simulink model "SecRwRtStLgrstInwdOtwdIsPosChk"  (R2024b)
settings: Solver=FixedStepDiscrete  StartTime=0.0  StopTime=10.0  FixedStep=0.01  RelTol=1e-3
undefined symbols (not defined in the file or in its folder): KeSMSuSecRwStLegrestInOutPosDelta_Val, KeSMSuSecRwStLegrestInOutPosTolr_Val
libraries: StIsPosChkLib x18, simulink x8
(part 1 of 2)
settings Model: Creator=sn2xws  LastModifiedBy=sn55gm
settings Model: ModifiedHistory=|
  | 2023.8.1 V2.0.0 CR421790 增加模式21-26
  | 2023.9.14 V2.1.0 Bug 540886 修改模式判断到位的条件为10ms周期计算
  | 2024.5.8 V3.0.0 557 eze 模式变更
  | 2024.7.9 V3.0.1 557模式流程V1.9
  | 2024.8.15 V3.0.2 智享模式需要计算目标位置，不能直接判断到位置，posalready赋值0
  | 2024.8.29 V3.0.3智享VIP目标位置用了4s问题修复
  | 2024.9.5 V3.0.4 新增Md56，注释不用的模式
  | 2024.10.14 V3.0.5 新增Md57，Md58
  | 2024.11.27 V3.0.6 Md57运行时，不能直接判断到位置
  | 25.7.7 V3.13.0 新增Md61 Md62 Md30 Md31
  | 25.10.30 V3.13.1 mode30标定修改
settings SolverCC: AlgebraicLoopSolver=TrustRegion
settings DataIOCC: SaveFormat=StructureWithTime  ReturnWorkspaceOutputs=off
settings OptimizationCC: DefaultParameterBehavior=Inlined  EnhancedBackFolding=on  PassReuseOutputArgsAs=Individual arguments  ZeroExternalMemoryAtStartup=off  ZeroInternalMemoryAtStartup=off  OptimizeBlockOrder=speed  DifferentSizesBufferReuse=on  OptimizationCustomize=off  EfficientTunableParamExpr=on
settings DebuggingCC: ParameterTunabilityLossMsg=error  UnconnectedInputMsg=warning  UnconnectedOutputMsg=warning  UnconnectedLineMsg=warning  ArithmeticOperatorsInVariantConditions=warning
settings ModelReferenceCC: EnableRefExpFcnMdlSchedulingChecks=on  ModelReferenceNumInstancesAllowed=Single
settings SFSimCC: MATLABDynamicMemAlloc=off  CustomCodeUndefinedFunction=UseInterfaceOnly
settings RTWCC: Description=AUTOSAR  SystemTargetFile=autosar.tlc  GenCodeOnly=on  TemplateMakefile=ert_default_tmf  GenerateReport=on  IncludeHyperlinkInReport=on  LaunchReport=on  DataTypeReplacement=CDataTypesFixedWidth  GenerateTraceInfo=on  GenerateTraceReport=on  GenerateTraceReportSl=on  GenerateTraceReportSf=on  GenerateTraceReportEml=on  GPUComputeCapability=3.5
settings CodeAppCC: ForceParamTrailComments=on  IgnoreCustomStorageClasses=off  OperatorAnnotations=on  SimulinkDataObjDesc=on  SFDataObjDesc=on  InsertBlockDesc=on
settings STFCustomTargetCC: TargetLangStandard=C99 (ISO)  MultiwordLength=256  ParMdlRefBuildCompliant=on  CompOptLevelCompliant=on  IncludeMdlTerminateFcn=off  CombineOutputUpdateFcns=on  SuppressErrorStatus=on  ERTCustomFileBanners=on  SupportNonFinite=off  SupportComplex=off  SupportContinuousTime=off  SupportNonInlinedSFcns=off  RemoveResetFunc=on  MATLABClassNameForMDSCustomization=Simulink.SoftwareTarget.ERTCustomization  AutosarCompliant=on  UseToolchainInfoCompliant=on  LookupTableObjectStructAxisOrder=2,1,3,4,...  LUTObjectStructOrderEvenSpacing=Size,Table,Breakpoints  SystemTargetFile=autosar.tlc
settings ERTTargetCC: TargetLangStandard=C99 (ISO)  ConcurrentExecutionCompliant=off  IncludeMdlTerminateFcn=off  SuppressErrorStatus=on  SupportNonFinite=off  SupportComplex=off  ModelStepFunctionPrototypeControlCompliant=off  CPPClassGenCompliant=off  AutosarCompliant=on  LookupTableObjectStructAxisOrder=2,1,3,4,...  LUTObjectStructOrderEvenSpacing=Size,Table,Breakpoints  ERTCustomFileTemplate=example_file_process.tlc  ERTFilePackagingFormat=Compact  BooleanTrueId=TRUE  BooleanFalseId=FALSE  DynamicArrayContainerType=coder::array

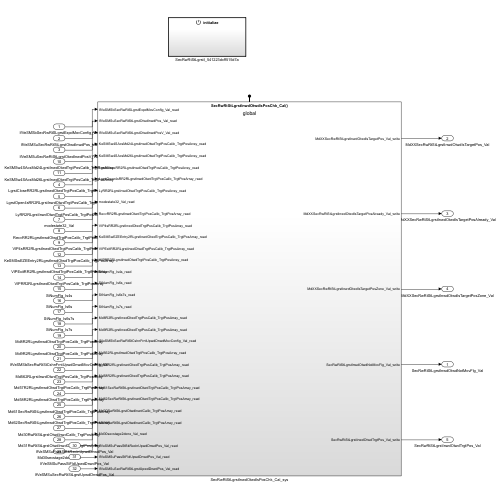
[thumbnail: Simulink's stored preview of the top-level diagram]
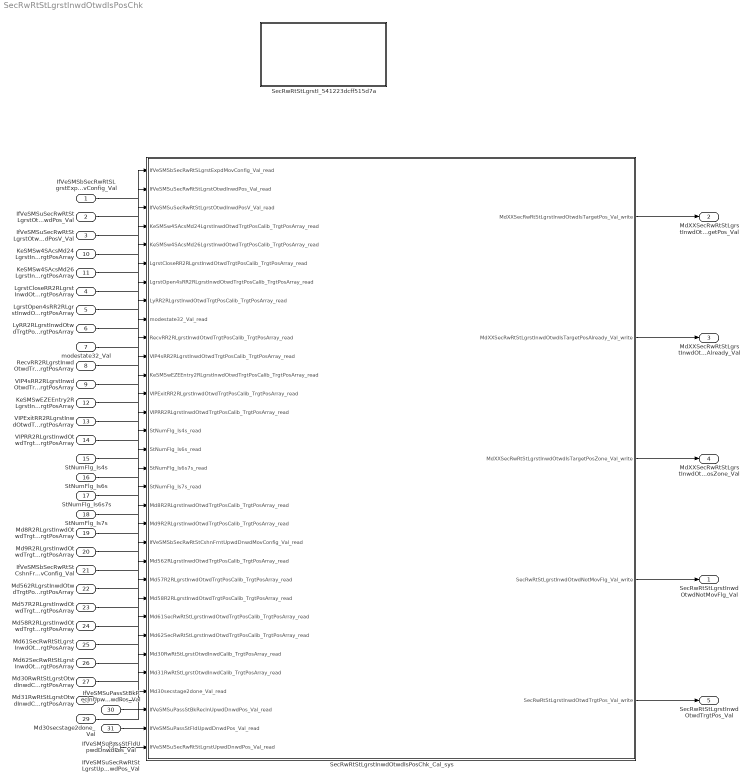
== system SecRwRtStLgrstInwdOtwdIsPosChk ==
  IfVeSMSbSecRwRtSLgrstExpdMovConfig_Val : Inport  OutDataTypeStr=boolean  PortDimensions=1
  IfVeSMSuSecRwRtStLgrstOtwdInwdPos_Val : Inport  Port=2  OutDataTypeStr=uint16  PortDimensions=1
  IfVeSMSuSecRwRtStLgrstOtwdInwdPosV_Val : Inport  Port=3  OutDataTypeStr=boolean  PortDimensions=1
  LgrstCloseRR2RLgrstInwdOtwdTrgtPosCalib_TrgtPosArray : Inport  Description=|  Port=4  OutDataTypeStr=uint16  PortDimensions=3
      | 0:Pos
      | 1:Max
      | 2:Min
  LgrstOpen4sRR2RLgrstInwdOtwdTrgtPosCalib_TrgtPosArray : Inport  Description=|  Port=5  OutDataTypeStr=uint16  PortDimensions=3
      | 0:Pos
      | 1:Max
      | 2:Min
  LyRR2RLgrstInwdOtwdTrgtPosCalib_TrgtPosArray : Inport  Description=|  Port=6  OutDataTypeStr=uint16  PortDimensions=3
      | 0:Pos
      | 1:Max
      | 2:Min
  modestate32_Val : Inport  Port=7  OutDataTypeStr=uint32  PortDimensions=1
  RecvRR2RLgrstInwdOtwdTrgtPosCalib_TrgtPosArray : Inport  Description=|  Port=8  OutDataTypeStr=uint16  PortDimensions=3
      | 0:Pos
      | 1:Max
      | 2:Min
  VIP4sRR2RLgrstInwdOtwdTrgtPosCalib_TrgtPosArray : Inport  Description=|  Port=9  OutDataTypeStr=uint16  PortDimensions=3
      | 0:Pos
      | 1:Max
      | 2:Min
  KeSMSw4SAcsMd24LgrstInwdOtwdTrgtPosCalib_TrgtPosArray : Inport  Description=|  Port=10  OutDataTypeStr=uint16  PortDimensions=3
      | 0:Pos
      | 1:Max
      | 2:Min
  KeSMSw4SAcsMd26LgrstInwdOtwdTrgtPosCalib_TrgtPosArray : Inport  Description=|  Port=11  OutDataTypeStr=uint16  PortDimensions=3
      | 0:Pos
      | 1:Max
      | 2:Min
  KeSMSwEZEEntry2RLgrstInwdOtwdTrgtPosCalib_TrgtPosArray : Inport  Description=|  Port=12  OutDataTypeStr=uint16  PortDimensions=3
      | 0:Pos
      | 1:Max
      | 2:Min
  VIPExitRR2RLgrstInwdOtwdTrgtPosCalib_TrgtPosArray : Inport  Description=|  Port=13  OutDataTypeStr=uint16  PortDimensions=3
      | 0:Pos
      | 1:Max
      | 2:Min
  VIPRR2RLgrstInwdOtwdTrgtPosCalib_TrgtPosArray : Inport  Description=|  Port=14  OutDataTypeStr=uint16  PortDimensions=3
      | 0:Pos
      | 1:Max
      | 2:Min
  StNumFlg_Is4s : Inport  Port=15  OutDataTypeStr=boolean  PortDimensions=1
  StNumFlg_Is6s : Inport  Port=16  OutDataTypeStr=boolean  PortDimensions=1
  StNumFlg_Is6s7s : Inport  Port=17  OutDataTypeStr=boolean  PortDimensions=1
  StNumFlg_Is7s : Inport  Port=18  OutDataTypeStr=boolean  PortDimensions=1
  Md8R2RLgrstInwdOtwdTrgtPosCalib_TrgtPosArray : Inport  Description=|  Port=19  OutDataTypeStr=uint16  PortDimensions=3
      | 0:Pos
      | 1:Max
      | 2:Min
  Md9R2RLgrstInwdOtwdTrgtPosCalib_TrgtPosArray : Inport  Description=|  Port=20  OutDataTypeStr=uint16  PortDimensions=3
      | 0:Pos
      | 1:Max
      | 2:Min
  IfVeSMSbSecRwRtStCshnFrntUpwdDnwdMovConfig_Val : Inport  Port=21  OutDataTypeStr=boolean  PortDimensions=1
  Md562RLgrstInwdOtwdTrgtPosCalib_TrgtPosArray : Inport  Description=|  Port=22  OutDataTypeStr=uint16  PortDimensions=3
      | 0:Pos
      | 1:Max
      | 2:Min
  Md57R2RLgrstInwdOtwdTrgtPosCalib_TrgtPosArray : Inport  Description=|  Port=23  OutDataTypeStr=uint16  PortDimensions=3
      | 0:Pos
      | 1:Max
      | 2:Min
  Md58R2RLgrstInwdOtwdTrgtPosCalib_TrgtPosArray : Inport  Description=|  Port=24  OutDataTypeStr=uint16  PortDimensions=3
      | 0:Pos
      | 1:Max
      | 2:Min
  Md61SecRwRtStLgrstInwdOtwdTrgtPosCalib_TrgtPosArray : Inport  Description=|  Port=25  OutDataTypeStr=uint16  PortDimensions=3
      | 0:Pos
      | 1:Max
      | 2:Min
  Md62SecRwRtStLgrstInwdOtwdTrgtPosCalib_TrgtPosArray : Inport  Description=|  Port=26  OutDataTypeStr=uint16  PortDimensions=3
      | 0:Pos
      | 1:Max
      | 2:Min
  Md30RwRtStLgrstOtwdInwdCalib_TrgtPosArray : Inport  Description=|  Port=27  OutDataTypeStr=uint16  PortDimensions=3
      | 0:Pos
      | 1:Max
      | 2:Min
  Md31RwRtStLgrstOtwdInwdCalib_TrgtPosArray : Inport  Description=|  Port=28  OutDataTypeStr=uint16  PortDimensions=3
      | 0:Pos
      | 1:Max
      | 2:Min
  Md30secstage2done_Val : Inport  Port=29  OutDataTypeStr=uint8  PortDimensions=1
  IfVeSMSuPassStBkReclnUpwdDnwdPos_Val : Inport  Port=30  OutDataTypeStr=uint16  PortDimensions=1
  IfVeSMSuPassStFldUpwdDnwdPos_Val : Inport  Port=31  OutDataTypeStr=uint16  PortDimensions=1
  IfVeSMSuSecRwRtStLgrstUpwdDnwdPos_Val : Inport  Port=32  OutDataTypeStr=uint16  PortDimensions=1
  SecRwRtStLgrstI_541223dcff515d7a : Subsystem
  SecRwRtStLgrstInwdOtwdIsPosChk_Cal_sys : Subsystem
  SecRwRtStLgrstInwdOtwdNotMovFlg_Val : Outport  OutDataTypeStr=boolean  PortDimensions=1  VectorParamsAs1DForOutWhenUnconnected=off
  MdXXSecRwRtStLgrstInwdOtwdIsTargetPos_Val : Outport  Port=2  OutDataTypeStr=uint32  PortDimensions=1  VectorParamsAs1DForOutWhenUnconnected=off
  MdXXSecRwRtStLgrstInwdOtwdIsTargetPosAlready_Val : Outport  Port=3  OutDataTypeStr=uint32  PortDimensions=1  VectorParamsAs1DForOutWhenUnconnected=off
  MdXXSecRwRtStLgrstInwdOtwdIsTargetPosZone_Val : Outport  Port=4  OutDataTypeStr=uint32  PortDimensions=1  VectorParamsAs1DForOutWhenUnconnected=off
  SecRwRtStLgrstInwdOtwdTrgtPos_Val : Outport  Port=5  OutDataTypeStr=uint16  PortDimensions=1  VectorParamsAs1DForOutWhenUnconnected=off
  wires:
  IfVeSMSbSecRwRtSLgrstExpdMovConfig_Val/1 -> SecRwRtStLgrstInwdOtwdIsPosChk_Cal_sys/1(IfVeSMSbSecRwRtSLgrstExpdMovConfig_Val_read)
  IfVeSMSuSecRwRtStLgrstOtwdInwdPos_Val/1 -> SecRwRtStLgrstInwdOtwdIsPosChk_Cal_sys/2(IfVeSMSuSecRwRtStLgrstOtwdInwdPos_Val_read)
  IfVeSMSuSecRwRtStLgrstOtwdInwdPosV_Val/1 -> SecRwRtStLgrstInwdOtwdIsPosChk_Cal_sys/3(IfVeSMSuSecRwRtStLgrstOtwdInwdPosV_Val_read)
  LgrstCloseRR2RLgrstInwdOtwdTrgtPosCalib_TrgtPosArray/1 -> SecRwRtStLgrstInwdOtwdIsPosChk_Cal_sys/6(LgrstCloseRR2RLgrstInwdOtwdTrgtPosCalib_TrgtPosArray_read)
  LgrstOpen4sRR2RLgrstInwdOtwdTrgtPosCalib_TrgtPosArray/1 -> SecRwRtStLgrstInwdOtwdIsPosChk_Cal_sys/7(LgrstOpen4sRR2RLgrstInwdOtwdTrgtPosCalib_TrgtPosArray_read)
  LyRR2RLgrstInwdOtwdTrgtPosCalib_TrgtPosArray/1 -> SecRwRtStLgrstInwdOtwdIsPosChk_Cal_sys/8(LyRR2RLgrstInwdOtwdTrgtPosCalib_TrgtPosArray_read)
  RecvRR2RLgrstInwdOtwdTrgtPosCalib_TrgtPosArray/1 -> SecRwRtStLgrstInwdOtwdIsPosChk_Cal_sys/10(RecvRR2RLgrstInwdOtwdTrgtPosCalib_TrgtPosArray_read)
  VIP4sRR2RLgrstInwdOtwdTrgtPosCalib_TrgtPosArray/1 -> SecRwRtStLgrstInwdOtwdIsPosChk_Cal_sys/11(VIP4sRR2RLgrstInwdOtwdTrgtPosCalib_TrgtPosArray_read)
  SecRwRtStLgrstInwdOtwdIsPosChk_Cal_sys/1(MdXXSecRwRtStLgrstInwdOtwdIsTargetPos_Val_write) -> MdXXSecRwRtStLgrstInwdOtwdIsTargetPos_Val/1
  SecRwRtStLgrstInwdOtwdIsPosChk_Cal_sys/2(MdXXSecRwRtStLgrstInwdOtwdIsTargetPosAlready_Val_write) -> MdXXSecRwRtStLgrstInwdOtwdIsTargetPosAlready_Val/1
  SecRwRtStLgrstInwdOtwdIsPosChk_Cal_sys/3(MdXXSecRwRtStLgrstInwdOtwdIsTargetPosZone_Val_write) -> MdXXSecRwRtStLgrstInwdOtwdIsTargetPosZone_Val/1
  SecRwRtStLgrstInwdOtwdIsPosChk_Cal_sys/4(SecRwRtStLgrstInwdOtwdNotMovFlg_Val_write) -> SecRwRtStLgrstInwdOtwdNotMovFlg_Val/1
  SecRwRtStLgrstInwdOtwdIsPosChk_Cal_sys/5(SecRwRtStLgrstInwdOtwdTrgtPos_Val_write) -> SecRwRtStLgrstInwdOtwdTrgtPos_Val/1
  KeSMSw4SAcsMd24LgrstInwdOtwdTrgtPosCalib_TrgtPosArray/1 -> SecRwRtStLgrstInwdOtwdIsPosChk_Cal_sys/4(KeSMSw4SAcsMd24LgrstInwdOtwdTrgtPosCalib_TrgtPosArray_read)
  KeSMSw4SAcsMd26LgrstInwdOtwdTrgtPosCalib_TrgtPosArray/1 -> SecRwRtStLgrstInwdOtwdIsPosChk_Cal_sys/5(KeSMSw4SAcsMd26LgrstInwdOtwdTrgtPosCalib_TrgtPosArray_read)
  modestate32_Val/1 -> SecRwRtStLgrstInwdOtwdIsPosChk_Cal_sys/9(modestate32_Val_read)
  KeSMSwEZEEntry2RLgrstInwdOtwdTrgtPosCalib_TrgtPosArray/1 -> SecRwRtStLgrstInwdOtwdIsPosChk_Cal_sys/12(KeSMSwEZEEntry2RLgrstInwdOtwdTrgtPosCalib_TrgtPosArray_read)
  VIPExitRR2RLgrstInwdOtwdTrgtPosCalib_TrgtPosArray/1 -> SecRwRtStLgrstInwdOtwdIsPosChk_Cal_sys/13(VIPExitRR2RLgrstInwdOtwdTrgtPosCalib_TrgtPosArray_read)
  VIPRR2RLgrstInwdOtwdTrgtPosCalib_TrgtPosArray/1 -> SecRwRtStLgrstInwdOtwdIsPosChk_Cal_sys/14(VIPRR2RLgrstInwdOtwdTrgtPosCalib_TrgtPosArray_read)
  StNumFlg_Is4s/1 -> SecRwRtStLgrstInwdOtwdIsPosChk_Cal_sys/15(StNumFlg_Is4s_read)
  StNumFlg_Is6s/1 -> SecRwRtStLgrstInwdOtwdIsPosChk_Cal_sys/16(StNumFlg_Is6s_read)
  StNumFlg_Is6s7s/1 -> SecRwRtStLgrstInwdOtwdIsPosChk_Cal_sys/17(StNumFlg_Is6s7s_read)
  StNumFlg_Is7s/1 -> SecRwRtStLgrstInwdOtwdIsPosChk_Cal_sys/18(StNumFlg_Is7s_read)
  Md8R2RLgrstInwdOtwdTrgtPosCalib_TrgtPosArray/1 -> SecRwRtStLgrstInwdOtwdIsPosChk_Cal_sys/19(Md8R2RLgrstInwdOtwdTrgtPosCalib_TrgtPosArray_read)
  Md9R2RLgrstInwdOtwdTrgtPosCalib_TrgtPosArray/1 -> SecRwRtStLgrstInwdOtwdIsPosChk_Cal_sys/20(Md9R2RLgrstInwdOtwdTrgtPosCalib_TrgtPosArray_read)
  IfVeSMSbSecRwRtStCshnFrntUpwdDnwdMovConfig_Val/1 -> SecRwRtStLgrstInwdOtwdIsPosChk_Cal_sys/21(IfVeSMSbSecRwRtStCshnFrntUpwdDnwdMovConfig_Val_read)
  Md562RLgrstInwdOtwdTrgtPosCalib_TrgtPosArray/1 -> SecRwRtStLgrstInwdOtwdIsPosChk_Cal_sys/22(Md562RLgrstInwdOtwdTrgtPosCalib_TrgtPosArray_read)
  Md57R2RLgrstInwdOtwdTrgtPosCalib_TrgtPosArray/1 -> SecRwRtStLgrstInwdOtwdIsPosChk_Cal_sys/23(Md57R2RLgrstInwdOtwdTrgtPosCalib_TrgtPosArray_read)
  Md58R2RLgrstInwdOtwdTrgtPosCalib_TrgtPosArray/1 -> SecRwRtStLgrstInwdOtwdIsPosChk_Cal_sys/24(Md58R2RLgrstInwdOtwdTrgtPosCalib_TrgtPosArray_read)
  Md61SecRwRtStLgrstInwdOtwdTrgtPosCalib_TrgtPosArray/1 -> SecRwRtStLgrstInwdOtwdIsPosChk_Cal_sys/25(Md61SecRwRtStLgrstInwdOtwdTrgtPosCalib_TrgtPosArray_read)
  Md62SecRwRtStLgrstInwdOtwdTrgtPosCalib_TrgtPosArray/1 -> SecRwRtStLgrstInwdOtwdIsPosChk_Cal_sys/26(Md62SecRwRtStLgrstInwdOtwdTrgtPosCalib_TrgtPosArray_read)
  Md30RwRtStLgrstOtwdInwdCalib_TrgtPosArray/1 -> SecRwRtStLgrstInwdOtwdIsPosChk_Cal_sys/27(Md30RwRtStLgrstOtwdInwdCalib_TrgtPosArray_read)
  Md31RwRtStLgrstOtwdInwdCalib_TrgtPosArray/1 -> SecRwRtStLgrstInwdOtwdIsPosChk_Cal_sys/28(Md31RwRtStLgrstOtwdInwdCalib_TrgtPosArray_read)
  Md30secstage2done_Val/1 -> SecRwRtStLgrstInwdOtwdIsPosChk_Cal_sys/29(Md30secstage2done_Val_read)
  IfVeSMSuPassStBkReclnUpwdDnwdPos_Val/1 -> SecRwRtStLgrstInwdOtwdIsPosChk_Cal_sys/30(IfVeSMSuPassStBkReclnUpwdDnwdPos_Val_read)
  IfVeSMSuPassStFldUpwdDnwdPos_Val/1 -> SecRwRtStLgrstInwdOtwdIsPosChk_Cal_sys/31(IfVeSMSuPassStFldUpwdDnwdPos_Val_read)
  IfVeSMSuSecRwRtStLgrstUpwdDnwdPos_Val/1 -> SecRwRtStLgrstInwdOtwdIsPosChk_Cal_sys/32(IfVeSMSuSecRwRtStLgrstUpwdDnwdPos_Val_read)

== system SecRwRtStLgrstInwdOtwdIsPosChk/SecRwRtStLgrstI_541223dcff515d7a ==
  note: Added blocks
  note: Added blocks
  Event Listener : EventListener  EventName=reset
  PA_KeSMSuSecRwStLegrestInOutPosDelta_Val : Constant  Value=KeSMSuSecRwStLegrestInOutPosDelta_Val
  PA_KeSMSuSecRwStLegrestInOutPosTolr_Val : Constant  Value=KeSMSuSecRwStLegrestInOutPosTolr_Val
  Terminator_1 : Terminator
  Terminator_2 : Terminator
  wires:
  PA_KeSMSuSecRwStLegrestInOutPosDelta_Val/1 -> Terminator_1/1
  PA_KeSMSuSecRwStLegrestInOutPosTolr_Val/1 -> Terminator_2/1

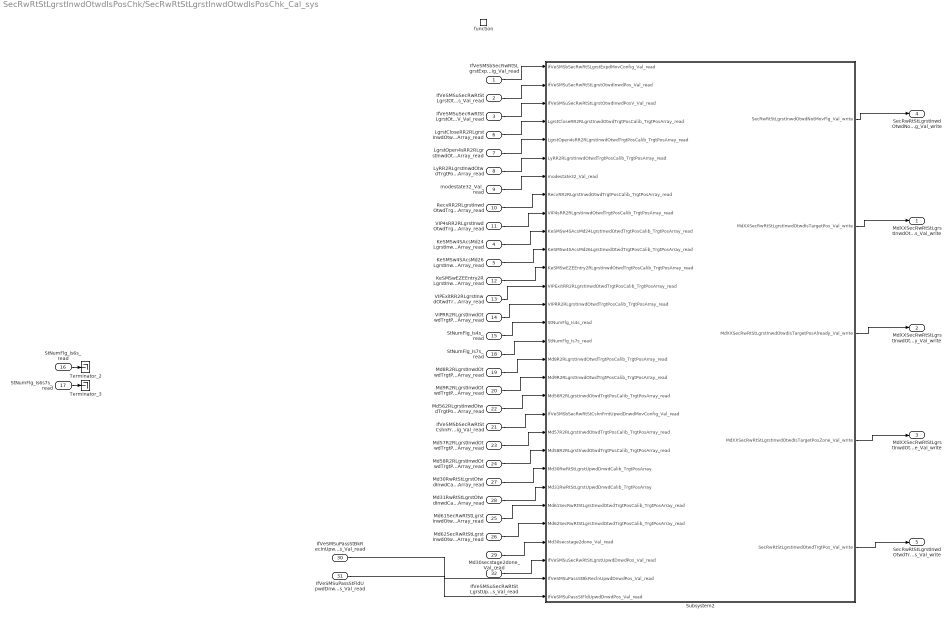
== system SecRwRtStLgrstInwdOtwdIsPosChk/SecRwRtStLgrstInwdOtwdIsPosChk_Cal_sys ==
  IfVeSMSbSecRwRtSLgrstExpdMovConfig_Val_read : Inport
  IfVeSMSuSecRwRtStLgrstOtwdInwdPos_Val_read : Inport  Port=2
  IfVeSMSuSecRwRtStLgrstOtwdInwdPosV_Val_read : Inport  Port=3
  KeSMSw4SAcsMd24LgrstInwdOtwdTrgtPosCalib_TrgtPosArray_read : Inport  Port=4
  KeSMSw4SAcsMd26LgrstInwdOtwdTrgtPosCalib_TrgtPosArray_read : Inport  Port=5
  LgrstCloseRR2RLgrstInwdOtwdTrgtPosCalib_TrgtPosArray_read : Inport  Port=6
  LgrstOpen4sRR2RLgrstInwdOtwdTrgtPosCalib_TrgtPosArray_read : Inport  Port=7
  LyRR2RLgrstInwdOtwdTrgtPosCalib_TrgtPosArray_read : Inport  Port=8
  modestate32_Val_read : Inport  Port=9
  RecvRR2RLgrstInwdOtwdTrgtPosCalib_TrgtPosArray_read : Inport  Port=10
  VIP4sRR2RLgrstInwdOtwdTrgtPosCalib_TrgtPosArray_read : Inport  Port=11
  KeSMSwEZEEntry2RLgrstInwdOtwdTrgtPosCalib_TrgtPosArray_read : Inport  Port=12
  VIPExitRR2RLgrstInwdOtwdTrgtPosCalib_TrgtPosArray_read : Inport  Port=13
  VIPRR2RLgrstInwdOtwdTrgtPosCalib_TrgtPosArray_read : Inport  Port=14
  StNumFlg_Is4s_read : Inport  Port=15
  StNumFlg_Is6s_read : Inport  Port=16
  StNumFlg_Is6s7s_read : Inport  Port=17
  StNumFlg_Is7s_read : Inport  Port=18
  Md8R2RLgrstInwdOtwdTrgtPosCalib_TrgtPosArray_read : Inport  Port=19
  Md9R2RLgrstInwdOtwdTrgtPosCalib_TrgtPosArray_read : Inport  Port=20
  IfVeSMSbSecRwRtStCshnFrntUpwdDnwdMovConfig_Val_read : Inport  Port=21
  Md562RLgrstInwdOtwdTrgtPosCalib_TrgtPosArray_read : Inport  Port=22
  Md57R2RLgrstInwdOtwdTrgtPosCalib_TrgtPosArray_read : Inport  Port=23
  Md58R2RLgrstInwdOtwdTrgtPosCalib_TrgtPosArray_read : Inport  Port=24
  Md61SecRwRtStLgrstInwdOtwdTrgtPosCalib_TrgtPosArray_read : Inport  Port=25
  Md62SecRwRtStLgrstInwdOtwdTrgtPosCalib_TrgtPosArray_read : Inport  Port=26
  Md30RwRtStLgrstOtwdInwdCalib_TrgtPosArray_read : Inport  Port=27
  Md31RwRtStLgrstOtwdInwdCalib_TrgtPosArray_read : Inport  Port=28
  Md30secstage2done_Val_read : Inport  Port=29
  IfVeSMSuPassStBkReclnUpwdDnwdPos_Val_read : Inport  Port=30
  IfVeSMSuPassStFldUpwdDnwdPos_Val_read : Inport  Port=31
  IfVeSMSuSecRwRtStLgrstUpwdDnwdPos_Val_read : Inport  Port=32
  function : TriggerPort  TriggerType=function-call  IsSimulinkFunction=on  FunctionName=SecRwRtStLgrstInwdOtwdIsPosChk_Cal  VariantControl=(inherit)
  Subsystem2 : Subsystem
  Terminator_2 : Terminator
  Terminator_3 : Terminator
  MdXXSecRwRtStLgrstInwdOtwdIsTargetPos_Val_write : Outport  VectorParamsAs1DForOutWhenUnconnected=off
      settings: EnsureOutportIsVirtual=on
  MdXXSecRwRtStLgrstInwdOtwdIsTargetPosAlready_Val_write : Outport  Port=2  VectorParamsAs1DForOutWhenUnconnected=off
      settings: EnsureOutportIsVirtual=on
  MdXXSecRwRtStLgrstInwdOtwdIsTargetPosZone_Val_write : Outport  Port=3  VectorParamsAs1DForOutWhenUnconnected=off
      settings: EnsureOutportIsVirtual=on
  SecRwRtStLgrstInwdOtwdNotMovFlg_Val_write : Outport  Port=4  VectorParamsAs1DForOutWhenUnconnected=off
      settings: EnsureOutportIsVirtual=on
  SecRwRtStLgrstInwdOtwdTrgtPos_Val_write : Outport  Port=5  VectorParamsAs1DForOutWhenUnconnected=off
      settings: EnsureOutportIsVirtual=on
  wires:
  Subsystem2/1(SecRwRtStLgrstInwdOtwdNotMovFlg_Val_write) -> SecRwRtStLgrstInwdOtwdNotMovFlg_Val_write/1
  Subsystem2/2(MdXXSecRwRtStLgrstInwdOtwdIsTargetPos_Val_write) -> MdXXSecRwRtStLgrstInwdOtwdIsTargetPos_Val_write/1
  Subsystem2/3(MdXXSecRwRtStLgrstInwdOtwdIsTargetPosAlready_Val_write) -> MdXXSecRwRtStLgrstInwdOtwdIsTargetPosAlready_Val_write/1
  Subsystem2/4(MdXXSecRwRtStLgrstInwdOtwdIsTargetPosZone_Val_write) -> MdXXSecRwRtStLgrstInwdOtwdIsTargetPosZone_Val_write/1
  Subsystem2/5(SecRwRtStLgrstInwdOtwdTrgtPos_Val_write) -> SecRwRtStLgrstInwdOtwdTrgtPos_Val_write/1
  VIP4sRR2RLgrstInwdOtwdTrgtPosCalib_TrgtPosArray_read/1 -> Subsystem2/9(VIP4sRR2RLgrstInwdOtwdTrgtPosCalib_TrgtPosArray_read)
  modestate32_Val_read/1 -> Subsystem2/7(modestate32_Val_read)
  RecvRR2RLgrstInwdOtwdTrgtPosCalib_TrgtPosArray_read/1 -> Subsystem2/8(RecvRR2RLgrstInwdOtwdTrgtPosCalib_TrgtPosArray_read)
  KeSMSw4SAcsMd24LgrstInwdOtwdTrgtPosCalib_TrgtPosArray_read/1 -> Subsystem2/10(KeSMSw4SAcsMd24LgrstInwdOtwdTrgtPosCalib_TrgtPosArray_read)
  KeSMSw4SAcsMd26LgrstInwdOtwdTrgtPosCalib_TrgtPosArray_read/1 -> Subsystem2/11(KeSMSw4SAcsMd26LgrstInwdOtwdTrgtPosCalib_TrgtPosArray_read)
  IfVeSMSbSecRwRtSLgrstExpdMovConfig_Val_read/1 -> Subsystem2/1(IfVeSMSbSecRwRtSLgrstExpdMovConfig_Val_read)
  IfVeSMSuSecRwRtStLgrstOtwdInwdPos_Val_read/1 -> Subsystem2/2(IfVeSMSuSecRwRtStLgrstOtwdInwdPos_Val_read)
  IfVeSMSuSecRwRtStLgrstOtwdInwdPosV_Val_read/1 -> Subsystem2/3(IfVeSMSuSecRwRtStLgrstOtwdInwdPosV_Val_read)
  LgrstCloseRR2RLgrstInwdOtwdTrgtPosCalib_TrgtPosArray_read/1 -> Subsystem2/4(LgrstCloseRR2RLgrstInwdOtwdTrgtPosCalib_TrgtPosArray_read)
  LgrstOpen4sRR2RLgrstInwdOtwdTrgtPosCalib_TrgtPosArray_read/1 -> Subsystem2/5(LgrstOpen4sRR2RLgrstInwdOtwdTrgtPosCalib_TrgtPosArray_read)
  LyRR2RLgrstInwdOtwdTrgtPosCalib_TrgtPosArray_read/1 -> Subsystem2/6(LyRR2RLgrstInwdOtwdTrgtPosCalib_TrgtPosArray_read)
  KeSMSwEZEEntry2RLgrstInwdOtwdTrgtPosCalib_TrgtPosArray_read/1 -> Subsystem2/12(KeSMSwEZEEntry2RLgrstInwdOtwdTrgtPosCalib_TrgtPosArray_read)
  VIPExitRR2RLgrstInwdOtwdTrgtPosCalib_TrgtPosArray_read/1 -> Subsystem2/13(VIPExitRR2RLgrstInwdOtwdTrgtPosCalib_TrgtPosArray_read)
  VIPRR2RLgrstInwdOtwdTrgtPosCalib_TrgtPosArray_read/1 -> Subsystem2/14(VIPRR2RLgrstInwdOtwdTrgtPosCalib_TrgtPosArray_read)
  StNumFlg_Is4s_read/1 -> Subsystem2/15(StNumFlg_Is4s_read)
  StNumFlg_Is6s_read/1 -> Terminator_2/1
  StNumFlg_Is6s7s_read/1 -> Terminator_3/1
  StNumFlg_Is7s_read/1 -> Subsystem2/16(StNumFlg_Is7s_read)
  Md9R2RLgrstInwdOtwdTrgtPosCalib_TrgtPosArray_read/1 -> Subsystem2/18(Md9R2RLgrstInwdOtwdTrgtPosCalib_TrgtPosArray_read)
  Md8R2RLgrstInwdOtwdTrgtPosCalib_TrgtPosArray_read/1 -> Subsystem2/17(Md8R2RLgrstInwdOtwdTrgtPosCalib_TrgtPosArray_read)
  Md562RLgrstInwdOtwdTrgtPosCalib_TrgtPosArray_read/1 -> Subsystem2/19(Md56R2RLgrstInwdOtwdTrgtPosCalib_TrgtPosArray_read)
  IfVeSMSbSecRwRtStCshnFrntUpwdDnwdMovConfig_Val_read/1 -> Subsystem2/20(IfVeSMSbSecRwRtStCshnFrntUpwdDnwdMovConfig_Val_read)
  Md57R2RLgrstInwdOtwdTrgtPosCalib_TrgtPosArray_read/1 -> Subsystem2/21(Md57R2RLgrstInwdOtwdTrgtPosCalib_TrgtPosArray_read)
  Md58R2RLgrstInwdOtwdTrgtPosCalib_TrgtPosArray_read/1 -> Subsystem2/22(Md58R2RLgrstInwdOtwdTrgtPosCalib_TrgtPosArray_read)
  Md30RwRtStLgrstOtwdInwdCalib_TrgtPosArray_read/1 -> Subsystem2/23(Md30RwRtStLgrstUpwdDnwdCalib_TrgtPosArray)
  Md31RwRtStLgrstOtwdInwdCalib_TrgtPosArray_read/1 -> Subsystem2/24(Md31RwRtStLgrstUpwdDnwdCalib_TrgtPosArray)
  Md61SecRwRtStLgrstInwdOtwdTrgtPosCalib_TrgtPosArray_read/1 -> Subsystem2/25(Md61SecRwRtStLgrstInwdOtwdTrgtPosCalib_TrgtPosArray_read)
  Md62SecRwRtStLgrstInwdOtwdTrgtPosCalib_TrgtPosArray_read/1 -> Subsystem2/26(Md62SecRwRtStLgrstInwdOtwdTrgtPosCalib_TrgtPosArray_read)
  Md30secstage2done_Val_read/1 -> Subsystem2/27(Md30secstage2done_Val_read)
  IfVeSMSuPassStBkReclnUpwdDnwdPos_Val_read/1 -> Subsystem2/29(IfVeSMSuPassStBkReclnUpwdDnwdPos_Val_read)
  IfVeSMSuPassStFldUpwdDnwdPos_Val_read/1 -> Subsystem2/30(IfVeSMSuPassStFldUpwdDnwdPos_Val_read)
  IfVeSMSuSecRwRtStLgrstUpwdDnwdPos_Val_read/1 -> Subsystem2/28(IfVeSMSuSecRwRtStLgrstUpwdDnwdPos_Val_read)

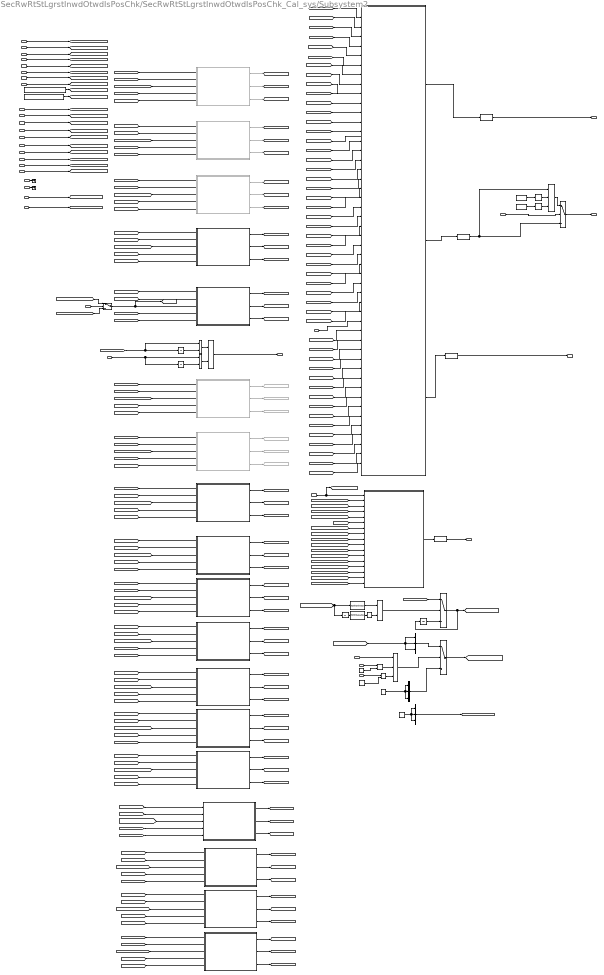
== system SecRwRtStLgrstInwdOtwdIsPosChk/SecRwRtStLgrstInwdOtwdIsPosChk_Cal_sys/Subsystem2 ==
  note: 2023.9.14 V2.1.0 Bug 540886 修改模式判断到位的条件为10ms周期计算
  note: 2023.8.1 V2.0.0 CR421790 增加模式21-26
  IfVeSMSbSecRwRtSLgrstExpdMovConfig_Val_read : Inport
  IfVeSMSuSecRwRtStLgrstOtwdInwdPos_Val_read : Inport  Port=2
  IfVeSMSuSecRwRtStLgrstOtwdInwdPosV_Val_read : Inport  Port=3
  LgrstCloseRR2RLgrstInwdOtwdTrgtPosCalib_TrgtPosArray_read : Inport  Port=4
  LgrstOpen4sRR2RLgrstInwdOtwdTrgtPosCalib_TrgtPosArray_read : Inport  Port=5
  LyRR2RLgrstInwdOtwdTrgtPosCalib_TrgtPosArray_read : Inport  Port=6
  modestate32_Val_read : Inport  Port=7
  RecvRR2RLgrstInwdOtwdTrgtPosCalib_TrgtPosArray_read : Inport  Port=8
  VIP4sRR2RLgrstInwdOtwdTrgtPosCalib_TrgtPosArray_read : Inport  Port=9
  KeSMSw4SAcsMd24LgrstInwdOtwdTrgtPosCalib_TrgtPosArray_read : Inport  Port=10
  KeSMSw4SAcsMd26LgrstInwdOtwdTrgtPosCalib_TrgtPosArray_read : Inport  Port=11
  KeSMSwEZEEntry2RLgrstInwdOtwdTrgtPosCalib_TrgtPosArray_read : Inport  Port=12
  VIPExitRR2RLgrstInwdOtwdTrgtPosCalib_TrgtPosArray_read : Inport  Port=13
  VIPRR2RLgrstInwdOtwdTrgtPosCalib_TrgtPosArray_read : Inport  Port=14
  StNumFlg_Is4s_read : Inport  Port=15
  StNumFlg_Is7s_read : Inport  Port=16
  Md8R2RLgrstInwdOtwdTrgtPosCalib_TrgtPosArray_read : Inport  Port=17
  Md9R2RLgrstInwdOtwdTrgtPosCalib_TrgtPosArray_read : Inport  Port=18
  Md56R2RLgrstInwdOtwdTrgtPosCalib_TrgtPosArray_read : Inport  Port=19
  IfVeSMSbSecRwRtStCshnFrntUpwdDnwdMovConfig_Val_read : Inport  Port=20
  Md57R2RLgrstInwdOtwdTrgtPosCalib_TrgtPosArray_read : Inport  Port=21
  Md58R2RLgrstInwdOtwdTrgtPosCalib_TrgtPosArray_read : Inport  Port=22
  Md30RwRtStLgrstUpwdDnwdCalib_TrgtPosArray : Inport  Port=23
  Md31RwRtStLgrstUpwdDnwdCalib_TrgtPosArray : Inport  Port=24
  Md61SecRwRtStLgrstInwdOtwdTrgtPosCalib_TrgtPosArray_read : Inport  Port=25
  Md62SecRwRtStLgrstInwdOtwdTrgtPosCalib_TrgtPosArray_read : Inport  Port=26
  Md30secstage2done_Val_read : Inport  Port=27
  IfVeSMSuSecRwRtStLgrstUpwdDnwdPos_Val_read : Inport  Port=28
  IfVeSMSuPassStBkReclnUpwdDnwdPos_Val_read : Inport  Port=29
  IfVeSMSuPassStFldUpwdDnwdPos_Val_read : Inport  Port=30
  32BitSelector1 : StIsPosChkLib/32BitSelector  BitNum=29
  32BitSelector14 : StIsPosChkLib/32BitSelector  BitNum=29
  Bitwise Operator : simulink/Logic and Bit Operations/Bitwise Operator  logicop=AND  UseBitMask=off  NumInputPorts=3  BitMask=bin2dec('11011001')  BitMaskRealWorld=Stored Integer
  Bitwise Operator1 : simulink/Logic and Bit Operations/Bitwise Operator  logicop=NOT  UseBitMask=off  BitMask=bin2dec('11011001')  BitMaskRealWorld=Stored Integer
  Bitwise Operator2 : simulink/Logic and Bit Operations/Bitwise Operator  logicop=NOT  UseBitMask=off  BitMask=bin2dec('11011001')  BitMaskRealWorld=Stored Integer
  Constant : Constant  Value=2048  OutDataTypeStr=uint32
  Constant1 : Constant  Value=1048576  OutDataTypeStr=uint32
  Constant10 : Constant  Value=0  OutDataTypeStr=uint16
  Constant2 : Constant  Value=120
  Constant3 : Constant  Value=120
  Constant9 : Constant  Value=0  OutDataTypeStr=uint16
  Data Type Conversion{,1..3} (4 alike) : DataTypeConversion  SaturateOnIntegerOverflow=off  RndMeth=Floor
  Goto28 : Goto  Commented=on  GotoTag=Md24IsTargetPosAlready
  Goto29 : Goto  Commented=on  GotoTag=Md24IsTargetPos
  Goto30 : Goto  Commented=on  GotoTag=Md24IsTargetPosZone
  Goto31 : Goto  Commented=on  GotoTag=Md26IsTargetPosAlready
  Goto32 : Goto  Commented=on  GotoTag=Md26IsTargetPos
  Goto33 : Goto  Commented=on  GotoTag=Md26IsTargetPosZone
  Logical Operator : Logic  AllPortsSameDT=off  OutDataTypeStr=boolean
  Logical Operator1 : Logic  Operator=NOT  AllPortsSameDT=off  OutDataTypeStr=boolean
  Logical Operator2 : Logic  AllPortsSameDT=off  OutDataTypeStr=boolean
  Logical Operator3 : Logic  Inputs=3  AllPortsSameDT=off  OutDataTypeStr=boolean
  Mux1 : Mux  Inputs=3
  Mux6 : Mux  Inputs=3
  Mux7 : Mux  Inputs=3
  PA_KeSMSuSecRwStLegrestInOutPosDelta_Val : Constant  Value=KeSMSuSecRwStLegrestInOutPosDelta_Val
  PA_KeSMSuSecRwStLegrestInOutPosTolr_Val : Constant  Value=KeSMSuSecRwStLegrestInOutPosTolr_Val
  Relational Operator : RelationalOperator  Operator===  OutDataTypeStr=boolean  RndMeth=Simplest  InputSameDT=off
  Relational Operator1 : RelationalOperator  Operator===  OutDataTypeStr=boolean  RndMeth=Simplest  InputSameDT=off
  Relational Operator2 : RelationalOperator  Operator=<=  OutDataTypeStr=boolean  RndMeth=Simplest  InputSameDT=off
  Relational Operator3 : RelationalOperator  Operator=<=  OutDataTypeStr=boolean  RndMeth=Simplest  InputSameDT=off
  Subsystem : Subsystem
  Subsystem1 : Subsystem
  Subsystem10 : Subsystem
  Subsystem11 : Subsystem
  Subsystem12 : Subsystem
  Subsystem13 : Subsystem
  Subsystem14 : Subsystem
  Subsystem15 : Subsystem
  Subsystem16 : Subsystem
  Subsystem17 : Subsystem
  Subsystem18 : Subsystem
  Subsystem19 : Subsystem
  Subsystem2 : Subsystem  Commented=on
  Subsystem3 : Subsystem  Commented=on
  Subsystem4 : Subsystem  Commented=on
  Subsystem5 : Subsystem
  Subsystem6 : Subsystem
  Subsystem7 : Subsystem  Commented=on
  Subsystem8 : Subsystem  Commented=on
  Subsystem9 : Subsystem
  Switch{,1..3} (4 alike) : Switch  Criteria=u2 > Threshold  SaturateOnIntegerOverflow=off  InputSameDT=off
  Terminator_1 : Terminator
  Terminator_2 : Terminator
  Unit Delay{,1..3} (4 alike) : UnitDelay  SampleTime=-1  HasFrameUpgradeWarning=on
  SecRwRtStLgrstInwdOtwdNotMovFlg_Val_write : Outport  VectorParamsAs1DForOutWhenUnconnected=off
      settings: EnsureOutportIsVirtual=on
  MdXXSecRwRtStLgrstInwdOtwdIsTargetPos_Val_write : Outport  Port=2  VectorParamsAs1DForOutWhenUnconnected=off
      settings: EnsureOutportIsVirtual=on
  MdXXSecRwRtStLgrstInwdOtwdIsTargetPosAlready_Val_write : Outport  Port=3  VectorParamsAs1DForOutWhenUnconnected=off
      settings: EnsureOutportIsVirtual=on
  MdXXSecRwRtStLgrstInwdOtwdIsTargetPosZone_Val_write : Outport  Port=4  VectorParamsAs1DForOutWhenUnconnected=off
      settings: EnsureOutportIsVirtual=on
  SecRwRtStLgrstInwdOtwdTrgtPos_Val_write : Outport  Port=5  VectorParamsAs1DForOutWhenUnconnected=off
      settings: EnsureOutportIsVirtual=on
  wires:
  [PosDelta] -> Subsystem6/4(Delta)
  Subsystem1/3(IsTargetPosZone) -> Data Type Conversion3/1
  Subsystem2/1(IsPos) -> [LgrstOpenLIsTargetPos]
  PA_KeSMSuSecRwStLegrestInOutPosTolr_Val/1 -> [PosTolr]
  [LgrstOpenLIsTargetPosAlready] -> Subsystem1/12(LgrstOpenLIsTargetPosAlready)
  [MovConfig] -> Subsystem1/7(MovConfig)
  [LgrstCloseLCalib] -> Subsystem/3(LgrstCloseLCalib)
  [PosV] -> Subsystem4/1(PosV)
  VIP4sRR2RLgrstInwdOtwdTrgtPosCalib_TrgtPosArray_read/1 -> [VIPLCalib]
  [RecvLCalib] -> Subsystem/5(RecvLCalib)
  IfVeSMSuSecRwRtStLgrstOtwdInwdPosV_Val_read/1 -> [PosV]
  RecvRR2RLgrstInwdOtwdTrgtPosCalib_TrgtPosArray_read/1 -> [RecvLCalib]
  IfVeSMSuSecRwRtStLgrstOtwdInwdPos_Val_read/1 -> [Pos]
  [LyLIsTargetPos] -> ?
  Subsystem1/2(IsTargetPosAlready) -> Data Type Conversion2/1
  [RecvLIsTargetPosZone] -> Subsystem1/19(RecvLIsTargetPosZone)
  [LyLCalib] -> Subsystem/4(LyLCalib)
  modestate32_Val_read/1 -> [modestate32_Val_read], Subsystem/1(modestate32_Val_read)
  Subsystem5/2(IsPosZone) -> [RecvLIsTargetPosZone]
  Subsystem1/1(IsTargetPos) -> Data Type Conversion1/1
  Subsystem3/3(IsPosAlready) -> [LgrstCloseLIsTargetPosAlready]
  LyRR2RLgrstInwdOtwdTrgtPosCalib_TrgtPosArray_read/1 -> [LyLCalib]
  PA_KeSMSuSecRwStLegrestInOutPosDelta_Val/1 -> [PosDelta]
  LgrstCloseRR2RLgrstInwdOtwdTrgtPosCalib_TrgtPosArray_read/1 -> [LgrstCloseLCalib]
  LgrstOpen4sRR2RLgrstInwdOtwdTrgtPosCalib_TrgtPosArray_read/1 -> [LgrstOpenLCalib]
  [Pos] -> Subsystem3/2(Pos)
  [LyLCalib] -> Subsystem4/3(CalibArray)
  [PosV] -> Subsystem3/1(PosV)
  IfVeSMSbSecRwRtSLgrstExpdMovConfig_Val_read/1 -> [MovConfig]
  Logical Operator2/1 -> SecRwRtStLgrstInwdOtwdNotMovFlg_Val_write/1
  [RecvLIsTargetPosAlready] -> Subsystem1/14(RecvLIsTargetPosAlready)
  [PosDelta] -> Subsystem2/4(Delta)
  Data Type Conversion1/1 -> MdXXSecRwRtStLgrstInwdOtwdIsTargetPos_Val_write/1
  [LgrstOpenLIsTargetPos] -> Subsystem1/8(LgrstOpenLIsTargetPos)
  [LgrstOpenLIsTargetPosZone] -> Subsystem1/16(LgrstOpenLIsTargetPosZone)
  [PosDelta] -> Subsystem4/4(Delta)
  Subsystem5/3(IsPosAlready) -> [RecvLIsTargetPosAlready]
  [PosDelta] -> Subsystem3/4(Delta)
  Subsystem6/1(IsPos) -> [VIPLIsTargetPos]
  [VIPL557Calib] -> Subsystem/6(VIPLCalib)
  [VIPLIsTargetPosZone] -> Subsystem1/20(VIPLIsTargetPosZone)
  Subsystem6/2(IsPosZone) -> [VIPLIsTargetPosZone]
  [Pos] -> Subsystem5/2(Pos)
  [PosTolr] -> Subsystem2/5(Tolr)
  [Pos] -> Subsystem2/2(Pos)
  [PosV] -> Subsystem5/1(PosV)
  [VIPLIsTargetPosAlready] -> Subsystem1/15(VIPLIsTargetPosAlready)
  Subsystem4/2(IsPosZone) -> [LyLIsTargetPosZone]
  Subsystem5/1(IsPos) -> [RecvLIsTargetPos]
  [PosTolr] -> Subsystem5/5(Tolr)
  Subsystem3/1(IsPos) -> [LgrstCloseLIsTargetPos]
  [LgrstCloseLIsTargetPosAlready] -> Subsystem1/13(LgrstCloseLIsTargetPosAlready)
  [LgrstCloseLIsTargetPosZone] -> Subsystem1/17(LgrstCloseLIsTargetPosZone)
  [RecvLIsTargetPos] -> Subsystem1/10(RecvLIsTargetPos)
  Subsystem/1(TrgtPos) -> Data Type Conversion/1
  Subsystem3/2(IsPosZone) -> [LgrstCloseLIsTargetPosZone]
  Subsystem4/3(IsPosAlready) -> [LyLIsTargetPosAlready]
  [Pos] -> Subsystem4/2(Pos)
  [LyLIsTargetPosZone] -> Subsystem1/18(LyLIsTargetPosZone)
  [PosV] -> Subsystem2/1(PosV)
  Subsystem6/3(IsPosAlready) -> [VIPLIsTargetPosAlready]
  [RecvLCalib] -> Subsystem5/3(CalibArray)
  [PosTolr] -> Subsystem4/5(Tolr)
  [VIPLIsTargetPos] -> Subsystem1/11(VIPLIsTargetPos)
  [PosV] -> Subsystem6/1(PosV)
  Data Type Conversion/1 -> SecRwRtStLgrstInwdOtwdTrgtPos_Val_write/1
  Subsystem2/3(IsPosAlready) -> [LgrstOpenLIsTargetPosAlready]
  [LyLIsTargetPosAlready] -> ?
  [Pos] -> Subsystem6/2(Pos)
  [PosTolr] -> Subsystem6/5(Tolr)
  [LgrstCloseLIsTargetPos] -> Subsystem1/9(LgrstCloseLIsTargetPos)
  Subsystem4/1(IsPos) -> [LyLIsTargetPos]
  [PosTolr] -> Subsystem3/5(Tolr)
  Subsystem2/2(IsPosZone) -> [LgrstOpenLIsTargetPosZone]
  [LgrstOpenLCalib] -> Subsystem/2(LgrstOpenLCalib)
  [PosDelta] -> Subsystem5/4(Delta)
  Data Type Conversion3/1 -> MdXXSecRwRtStLgrstInwdOtwdIsTargetPosZone_Val_write/1
  KeSMSw4SAcsMd24LgrstInwdOtwdTrgtPosCalib_TrgtPosArray_read/1 -> [Md24Calib]
  KeSMSw4SAcsMd26LgrstInwdOtwdTrgtPosCalib_TrgtPosArray_read/1 -> [Md26Calib]
  [Md24Calib] -> Subsystem7/3(CalibArray)
  [PosTolr] -> Subsystem7/5(Tolr)
  [Pos] -> Subsystem7/2(Pos)
  [PosV] -> Subsystem7/1(PosV)
  Subsystem7/3(IsPosAlready) -> Goto28/1
  Subsystem7/2(IsPosZone) -> Goto30/1
  Subsystem7/1(IsPos) -> Goto29/1
  [PosDelta] -> Subsystem7/4(Delta)
  [PosDelta] -> Subsystem8/4(Delta)
  Subsystem8/1(IsPos) -> Goto32/1
  Subsystem8/2(IsPosZone) -> Goto33/1
  Subsystem8/3(IsPosAlready) -> Goto31/1
  [PosV] -> Subsystem8/1(PosV)
  [Pos] -> Subsystem8/2(Pos)
  [PosTolr] -> Subsystem8/5(Tolr)
  [Md26Calib] -> Subsystem8/3(CalibArray)
  [Md57Calib] -> Subsystem/7(Md57Calib)
  [Md58Calib] -> Subsystem/8(Md58Calib)
  [Md57IsTargetPos] -> Subsystem1/21(Md57IsTargetPos)
  [Md58IsTargetPos] -> Subsystem1/22(Md58IsTargetPos)
  [Md57IsTargetPosAlready] -> Subsystem1/23(Md57IsTargetPosAlready)
  [Md58IsTargetPosAlready] -> Subsystem1/24(Md58IsTargetPosAlready)
  [Md57IsTargetPosZone] -> Subsystem1/25(Md57IsTargetPosZone)
  [Md58IsTargetPosZone] -> Subsystem1/26(Md58IsTargetPosZone)
  [LgrstOpenLCalib] -> Subsystem2/3(CalibArray)
  [LgrstCloseLCalib] -> Subsystem3/3(CalibArray)
  KeSMSwEZEEntry2RLgrstInwdOtwdTrgtPosCalib_TrgtPosArray_read/1 -> [Md1Calib]
  [Md1Calib] -> Subsystem9/3(CalibArray)
  [PosTolr] -> Subsystem9/5(Tolr)
  [Pos] -> Subsystem9/2(Pos)
  [PosV] -> Subsystem9/1(PosV)
  Subsystem9/3(IsPosAlready) -> [Md1IsTargetPosAlready]
  Subsystem9/2(IsPosZone) -> [Md1IsTargetPosZone]
  Subsystem9/1(IsPos) -> [Md1IsTargetPos]
  [PosDelta] -> Subsystem9/4(Delta)
  [Md1Calib] -> Subsystem/9(Md1Calib)
  [Md1IsTargetPos] -> Subsystem1/27(Md1IsTargetPos)
  [Md1IsTargetPosAlready] -> Subsystem1/28(Md1IsTargetPosAlready)
  [Md1IsTargetPosZone] -> Subsystem1/29(Md1IsTargetPosZone)
  VIPExitRR2RLgrstInwdOtwdTrgtPosCalib_TrgtPosArray_read/1 -> [Md28Calib]
  VIPRR2RLgrstInwdOtwdTrgtPosCalib_TrgtPosArray_read/1 -> [VIP6s7sCalib]
  [PosDelta] -> Subsystem10/4(Delta)
  Subsystem10/1(IsPos) -> [Md28IsTargetPos]
  Subsystem10/2(IsPosZone) -> [Md28IsTargetPosZone]
  Subsystem10/3(IsPosAlready) -> [Md28IsTargetPosAlready]
  [PosV] -> Subsystem10/1(PosV)
  [Pos] -> Subsystem10/2(Pos)
  [PosTolr] -> Subsystem10/5(Tolr)
  [Md28Calib] -> Subsystem10/3(CalibArray)
  Switch/1 -> [VIPL557Calib], Subsystem6/3(CalibArray)
  [VIPLCalib] -> Switch/1
  StNumFlg_Is4s_read/1 -> Switch/2
  [VIP6s7sCalib] -> Switch/3
  [Md28Calib] -> Subsystem/10(Md28Calib)
  [Md28IsTargetPos] -> Subsystem1/30(Md28IsTargetPos)
  [Md28IsTargetPosAlready] -> Subsystem1/31(Md28IsTargetPosAlready)
  [Md28IsTargetPosZone] -> Subsystem1/32(Md28IsTargetPosZone)
  StNumFlg_Is7s_read/1 -> Subsystem1/33(StNumFlg_Is7s_read)
  Md8R2RLgrstInwdOtwdTrgtPosCalib_TrgtPosArray_read/1 -> [Md8Calib]
  Md9R2RLgrstInwdOtwdTrgtPosCalib_TrgtPosArray_read/1 -> [Md9Calib]
  Md56R2RLgrstInwdOtwdTrgtPosCalib_TrgtPosArray_read/1 -> [Md56Calib]
  [Md8Calib] -> Subsystem11/3(CalibArray)
  [PosTolr] -> Subsystem11/5(Tolr)
  [Pos] -> Subsystem11/2(Pos)
  [PosV] -> Subsystem11/1(PosV)
  Subsystem11/3(IsPosAlready) -> [Md8IsTargetPosAlready]
  Subsystem11/2(IsPosZone) -> [Md8IsTargetPosZone]
  Subsystem11/1(IsPos) -> [Md8IsTargetPos]
  [PosDelta] -> Subsystem11/4(Delta)
  [PosDelta] -> Subsystem12/4(Delta)
  Subsystem12/1(IsPos) -> [Md9IsTargetPos]
  Subsystem12/2(IsPosZone) -> [Md9IsTargetPosZone]
  Subsystem12/3(IsPosAlready) -> [Md9IsTargetPosAlready]
  [PosV] -> Subsystem12/1(PosV)
  [Pos] -> Subsystem12/2(Pos)
  [PosTolr] -> Subsystem12/5(Tolr)
  [Md9Calib] -> Subsystem12/3(CalibArray)
  [Md56Calib] -> Subsystem13/3(CalibArray)
  [PosTolr] -> Subsystem13/5(Tolr)
  [Pos] -> Subsystem13/2(Pos)
  [PosV] -> Subsystem13/1(PosV)
  Subsystem13/3(IsPosAlready) -> [Md56IsTargetPosAlready]
  Subsystem13/2(IsPosZone) -> [Md56IsTargetPosZone]
  Subsystem13/1(IsPos) -> [Md56IsTargetPos]
  [PosDelta] -> Subsystem13/4(Delta)
  [Md8Calib] -> Subsystem/11(Md8Calib)
  [Md9Calib] -> Subsystem/12(Md9Calib)
  [Md56Calib] -> Subsystem/13(Md56Calib)
  [Md8IsTargetPos] -> Subsystem1/34(Md8IsTargetPos)
  [Md9IsTargetPos] -> Subsystem1/35(Md9IsTargetPos)
  [Md56IsTargetPos] -> Subsystem1/36(Md56IsTargetPos)
  [Md8IsTargetPosAlready] -> Subsystem1/37(Md8IsTargetPosAlready)
  [Md9IsTargetPosAlready] -> Subsystem1/38(Md9IsTargetPosAlready)
  [Md56IsTargetPosAlready] -> Subsystem1/39(Md56IsTargetPosAlready)
  [Md8IsTargetPosZone] -> Subsystem1/40(Md8IsTargetPosZone)
  [Md9IsTargetPosZone] -> Subsystem1/41(Md9IsTargetPosZone)
  [Md56IsTargetPosZone] -> Subsystem1/42(Md56IsTargetPosZone)
  Constant/1 -> Bitwise Operator1/1
  Data Type Conversion2/1 -> Bitwise Operator/1, Switch1/3
  IfVeSMSbSecRwRtStCshnFrntUpwdDnwdMovConfig_Val_read/1 -> Switch1/2
  Switch1/1 -> MdXXSecRwRtStLgrstInwdOtwdIsTargetPosAlready_Val_write/1
  Bitwise Operator1/1 -> Bitwise Operator/2
  Bitwise Operator/1 -> Switch1/1
  Md58R2RLgrstInwdOtwdTrgtPosCalib_TrgtPosArray_read/1 -> [Md58Calib]
  Md57R2RLgrstInwdOtwdTrgtPosCalib_TrgtPosArray_read/1 -> [Md57Calib]
  [PosDelta] -> Subsystem14/4(Delta)
  Subsystem14/1(IsPos) -> [Md57IsTargetPos]
  Subsystem14/2(IsPosZone) -> [Md57IsTargetPosZone]
  Subsystem14/3(IsPosAlready) -> [Md57IsTargetPosAlready]
  [PosV] -> Subsystem14/1(PosV)
  [Pos] -> Subsystem14/2(Pos)
  [PosTolr] -> Subsystem14/5(Tolr)
  [Md57Calib] -> Subsystem14/3(CalibArray)
  [Md58Calib] -> Subsystem15/3(CalibArray)
  [PosTolr] -> Subsystem15/5(Tolr)
  [Pos] -> Subsystem15/2(Pos)
  [PosV] -> Subsystem15/1(PosV)
  Subsystem15/3(IsPosAlready) -> [Md58IsTargetPosAlready]
  Subsystem15/2(IsPosZone) -> [Md58IsTargetPosZone]
  Subsystem15/1(IsPos) -> [Md58IsTargetPos]
  [PosDelta] -> Subsystem15/4(Delta)
  Bitwise Operator2/1 -> Bitwise Operator/3
  Constant1/1 -> Bitwise Operator2/1
  [PosTolr] -> Subsystem17/5(Tolr)
  Subsystem17/2(IsPosZone) -> [Md30IsTargetPosZone]
  [PosDelta] -> Subsystem17/4(Delta)
  Subsystem18/1(IsPos) -> [Md31IsTargetPos]
  Subsystem18/2(IsPosZone) -> [Md31IsTargetPosZone]
  [Pos] -> Subsystem18/2(Pos)
  Subsystem17/1(IsPos) -> [Md30IsTargetPos]
  Subsystem18/3(IsPosAlready) -> [Md31IsTargetPosAlready]
  [Md30Calib] -> Subsystem17/3(CalibArray)
  [PosDelta] -> Subsystem18/4(Delta)
  [PosV] -> Subsystem18/1(PosV)
  [PosTolr] -> Subsystem18/5(Tolr)
  [PosV] -> Subsystem17/1(PosV)
  Subsystem17/3(IsPosAlready) -> [Md30IsTargetPosAlready]
  [Pos] -> Subsystem17/2(Pos)
  [Md31Calib] -> Subsystem18/3(CalibArray)
  [Md31IsTargetPosAlready] -> Subsystem1/6(Md31IsTargetPosAlready)
  [Md31IsTargetPosZone] -> Subsystem1/5(Md31IsTargetPosZone)
  [Md31IsTargetPos] -> Subsystem1/4(Md31IsTargetPos)
  [Md30IsTargetPosAlready] -> Subsystem1/3(Md30IsTargetPosAlready)
  [Md30IsTargetPosZone] -> Subsystem1/2(Md30IsTargetPosZone)
  [Md30IsTargetPos] -> Subsystem1/1(Md30IsTargetPos)
  [Md61Calib] -> Subsystem16/3(CalibArray)
  [PosTolr] -> Subsystem16/5(Tolr)
  [PosV] -> Subsystem16/1(PosV)
  [PosDelta] -> Subsystem16/4(Delta)
  Subsystem16/3(IsPosAlready) -> [Md61IsTargetPosAlready]
  [Pos] -> Subsystem16/2(Pos)
  Subsystem16/2(IsPosZone) -> [Md61IsTargetPosZone]
  Subsystem16/1(IsPos) -> [Md61IsTargetPos]
  Subsystem19/1(IsPos) -> [Md62IsTargetPos]
  Subsystem19/2(IsPosZone) -> [Md62IsTargetPosZone]
  [Pos] -> Subsystem19/2(Pos)
  Subsystem19/3(IsPosAlready) -> [Md62IsTargetPosAlready]
  [PosDelta] -> Subsystem19/4(Delta)
  [PosV] -> Subsystem19/1(PosV)
  [PosTolr] -> Subsystem19/5(Tolr)
  [Md62Calib] -> Subsystem19/3(CalibArray)
  [Md61IsTargetPos] -> Subsystem1/43(Md61IsTargetPos)
  [Md62IsTargetPos] -> Subsystem1/44(Md62IsTargetPos)
  [Md61IsTargetPosAlready] -> Subsystem1/45(Md61IsTargetPosAlready)
  [Md62IsTargetPosAlready] -> Subsystem1/46(Md62IsTargetPosAlready)
  [Md61IsTargetPosZone] -> Subsystem1/47(Md61IsTargetPosZone)
  [Md62IsTargetPosZone] -> Subsystem1/48(Md62IsTargetPosZone)
  [Md30Calib] -> Subsystem/14(Md30Calib)
  [Md31Calib] -> Subsystem/15(Md31Calib)
  [Md61Calib] -> Subsystem/16(Md61Calib)
  [Md62Calib] -> Subsystem/17(Md62Calib)
  Md61SecRwRtStLgrstInwdOtwdTrgtPosCalib_TrgtPosArray_read/1 -> [Md61Calib]
  Md62SecRwRtStLgrstInwdOtwdTrgtPosCalib_TrgtPosArray_read/1 -> [Md62Calib]
  [modestate32_Val_read] -> Unit Delay/1, 32BitSelector14/1
  Logical Operator/1 -> Switch2/2
  [Pos] -> Switch2/1
  Switch2/1 -> Unit Delay1/1, [LgrstOtWdInwdPosInit]
  32BitSelector14/1 -> Logical Operator/1
  32BitSelector1/1 -> Logical Operator1/1
  Logical Operator1/1 -> Logical Operator/2
  Unit Delay/1 -> 32BitSelector1/1
  Constant9/1 -> Mux7/1, Mux7/3, Mux7/2
  [LgrstOtWdInwdPosInit] -> Mux1/2, Mux1/3, Mux1/1
  Switch3/1 -> [Md30Calib]
  Mux6/1 -> [Md31Calib]
  Constant10/1 -> Mux6/1, Mux6/3, Mux6/2
  Md30RwRtStLgrstUpwdDnwdCalib_TrgtPosArray/1 -> Terminator_1/1
  Md31RwRtStLgrstUpwdDnwdCalib_TrgtPosArray/1 -> Terminator_2/1
  Unit Delay1/1 -> Switch2/3
  Mux1/1 -> Switch3/1
  Mux7/1 -> Switch3/3
  IfVeSMSuSecRwRtStLgrstUpwdDnwdPos_Val_read/1 -> Unit Delay3/1, Relational Operator1/1
  [Pos] -> Relational Operator/1, Unit Delay2/1
  Unit Delay3/1 -> Relational Operator1/2
  Unit Delay2/1 -> Relational Operator/2
  Relational Operator/1 -> Logical Operator2/1
  Relational Operator1/1 -> Logical Operator2/2
  Constant2/1 -> Relational Operator2/2
  IfVeSMSuPassStBkReclnUpwdDnwdPos_Val_read/1 -> Relational Operator2/1
  Constant3/1 -> Relational Operator3/2
  IfVeSMSuPassStFldUpwdDnwdPos_Val_read/1 -> Relational Operator3/1
  Relational Operator3/1 -> Logical Operator3/3
  Relational Operator2/1 -> Logical Operator3/2
  Md30secstage2done_Val_read/1 -> Logical Operator3/1
  Logical Operator3/1 -> Switch3/2

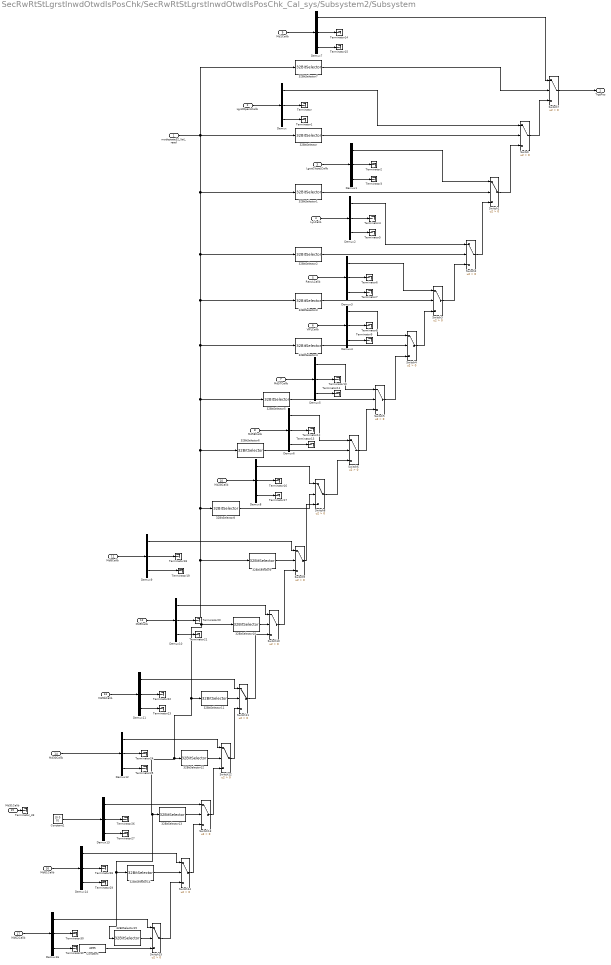
== system SecRwRtStLgrstInwdOtwdIsPosChk/SecRwRtStLgrstInwdOtwdIsPosChk_Cal_sys/Subsystem2/Subsystem ==
  modestate32_Val_read : Inport
  LgrstOpenLCalib : Inport  Port=2
  LgrstCloseLCalib : Inport  Port=3
  LyLCalib : Inport  Port=4
  RecvLCalib : Inport  Port=5
  VIPLCalib : Inport  Port=6
  Md57Calib : Inport  Port=7
  Md58Calib : Inport  Port=8
  Md1Calib : Inport  Port=9
  Md28Calib : Inport  Port=10
  Md8Calib : Inport  Port=11
  Md9Calib : Inport  Port=12
  Md56Calib : Inport  Port=13
  Md30Calib : Inport  Port=14
  Md31Calib : Inport  Port=15
  Md61Calib : Inport  Port=16
  Md62Calib : Inport  Port=17
  32BitSelector : StIsPosChkLib/32BitSelector  BitNum=17
  32BitSelector1 : StIsPosChkLib/32BitSelector  BitNum=18
  32BitSelector10 : StIsPosChkLib/32BitSelector  BitNum=8
  32BitSelector11 : StIsPosChkLib/32BitSelector  BitNum=24
  32BitSelector12 : StIsPosChkLib/32BitSelector  BitNum=29
  32BitSelector13 : StIsPosChkLib/32BitSelector  BitNum=30
  32BitSelector14 : StIsPosChkLib/32BitSelector  BitNum=5
  32BitSelector15 : StIsPosChkLib/32BitSelector  BitNum=6
  32BitSelector2 : StIsPosChkLib/32BitSelector  BitNum=14
  32BitSelector3 : StIsPosChkLib/32BitSelector  BitNum=12
  32BitSelector4 : StIsPosChkLib/32BitSelector  BitNum=11
  32BitSelector5 : StIsPosChkLib/32BitSelector  BitNum=20
  32BitSelector6 : StIsPosChkLib/32BitSelector  BitNum=21
  32BitSelector7 : StIsPosChkLib/32BitSelector  BitNum=0
  32BitSelector8 : StIsPosChkLib/32BitSelector  BitNum=27
  32BitSelector9 : StIsPosChkLib/32BitSelector  BitNum=7
  Constant : Constant  Value=4095  OutDataTypeStr=uint16
  Constant1 : Constant  Value=[0 0 0]
  Demux{,1..14,16} (16 alike) : Demux  Outputs=3
  Switch{,1..15} (16 alike) : Switch  Criteria=u2 > Threshold  SaturateOnIntegerOverflow=off  InputSameDT=off
  Terminator{,1..31} (32 alike) : Terminator
  Terminator_33 : Terminator
  TrgtPos : Outport  VectorParamsAs1DForOutWhenUnconnected=off
      settings: EnsureOutportIsVirtual=on
  wires:
  32BitSelector/1 -> Switch/2
  Demux/1 -> Switch/1
  Demux/3 -> Terminator1/1
  Demux/2 -> Terminator/1
  LgrstOpenLCalib/1 -> Demux/1
  LgrstCloseLCalib/1 -> Demux1/1
  Demux1/2 -> Terminator2/1
  Demux1/3 -> Terminator3/1
  Demux1/1 -> Switch1/1
  Switch1/1 -> Switch/3
  32BitSelector1/1 -> Switch1/2
  Switch2/1 -> Switch1/3
  Switch3/1 -> Switch2/3
  Switch4/1 -> Switch3/3
  32BitSelector2/1 -> Switch2/2
  32BitSelector3/1 -> Switch3/2
  32BitSelector4/1 -> Switch4/2
  Demux2/1 -> Switch2/1
  Demux2/3 -> Terminator5/1
  Demux2/2 -> Terminator4/1
  LyLCalib/1 -> Demux2/1
  RecvLCalib/1 -> Demux3/1
  Demux3/2 -> Terminator6/1
  Demux3/3 -> Terminator7/1
  Demux3/1 -> Switch3/1
  Demux4/1 -> Switch4/1
  Demux4/3 -> Terminator9/1
  Demux4/2 -> Terminator8/1
  VIPLCalib/1 -> Demux4/1
  Md57Calib/1 -> Demux5/1
  Demux5/2 -> Terminator10/1
  Demux5/3 -> Terminator11/1
  Demux5/1 -> Switch5/1
  32BitSelector5/1 -> Switch5/2
  32BitSelector6/1 -> Switch6/2
  Demux6/1 -> Switch6/1
  Demux6/3 -> Terminator13/1
  Demux6/2 -> Terminator12/1
  Md58Calib/1 -> Demux6/1
  Switch5/1 -> Switch4/3
  Switch6/1 -> Switch5/3
  Md1Calib/1 -> Demux7/1
  Demux7/2 -> Terminator14/1
  Demux7/3 -> Terminator15/1
  Demux7/1 -> Switch7/1
  Switch7/1 -> TrgtPos/1
  Switch/1 -> Switch7/3
  32BitSelector7/1 -> Switch7/2
  Switch8/1 -> Switch6/3
  32BitSelector8/1 -> Switch8/2
  Demux8/1 -> Switch8/1
  Demux8/2 -> Terminator16/1
  Demux8/3 -> Terminator17/1
  Md28Calib/1 -> Demux8/1
  modestate32_Val_read/1 -> 32BitSelector7/1, 32BitSelector/1, 32BitSelector1/1, 32BitSelector2/1, 32BitSelector3/1, 32BitSelector8/1, 32BitSelector9/1, 32BitSelector15/1, 32BitSelector14/1, 32BitSelector13/1, 32BitSelector12/1, 32BitSelector11/1, 32BitSelector10/1, 32BitSelector6/1, 32BitSelector5/1, 32BitSelector4/1
  Switch9/1 -> Switch8/3
  Switch10/1 -> Switch9/3
  Switch11/1 -> Switch10/3
  Md8Calib/1 -> Demux9/1
  Demux9/1 -> Switch9/1
  Demux9/2 -> Terminator18/1
  Demux9/3 -> Terminator19/1
  Demux10/3 -> Terminator21/1
  Demux10/2 -> Terminator20/1
  Demux10/1 -> Switch10/1
  Md9Calib/1 -> Demux10/1
  Md56Calib/1 -> Demux11/1
  Demux11/1 -> Switch11/1
  Demux11/2 -> Terminator22/1
  Demux11/3 -> Terminator23/1
  32BitSelector9/1 -> Switch9/2
  32BitSelector10/1 -> Switch10/2
  32BitSelector11/1 -> Switch11/2
  Switch12/1 -> Switch11/3
  Switch13/1 -> Switch12/3
  Switch14/1 -> Switch13/3
  Switch15/1 -> Switch14/3
  Constant/1 -> Switch15/3
  32BitSelector12/1 -> Switch12/2
  32BitSelector13/1 -> Switch13/2
  32BitSelector14/1 -> Switch14/2
  32BitSelector15/1 -> Switch15/2
  Demux12/3 -> Terminator25/1
  Demux12/2 -> Terminator24/1
  Demux12/1 -> Switch12/1
  Demux13/1 -> Switch13/1
  Demux13/2 -> Terminator26/1
  Demux13/3 -> Terminator27/1
  Demux14/3 -> Terminator29/1
  Demux14/2 -> Terminator28/1
  Demux14/1 -> Switch14/1
  Md61Calib/1 -> Demux14/1
  Md62Calib/1 -> Demux16/1
  Demux16/1 -> Switch15/1
  Demux16/2 -> Terminator30/1
  Demux16/3 -> Terminator31/1
  Md30Calib/1 -> Demux12/1
  Constant1/1 -> Demux13/1
  Md31Calib/1 -> Terminator_33/1
